simulink model "Nieliniowy"  (R2018a)
settings: Solver=ode45  StartTime=0.0  StopTime=200  RelTol=1e-3  AbsTol=1e-6  EnableMultiTasking=on
values from neighbouring files (symbols this model uses):
  A1 = 3500    [ZbiorniczkiLiniowe.m]
  A2 = 2000    [ZbiorniczkiLiniowe.m]
  Aw1 = 0.1 * A1    (= 350)    [ZbiorniczkiLiniowe.m]
  Aw2 = 0.1 * A2    (= 200)    [ZbiorniczkiLiniowe.m]
  df1 = 200    [ZbiorniczkiLiniowe.m]
  f1 = wektorf1(i)    [ZbiorniczkiLiniowe.m]
  g = 10    [ZbiorniczkiLiniowe.m]
  h1 = (f1/a1)+(f1+df2)/a2    [ZbiorniczkiLiniowe.m]
  h2 = (f1+df2)/a2    [ZbiorniczkiLiniowe.m]
  t1 = 40    [ZbiorniczkiLiniowe.m]
settings Model: Creator=LAB320-1552  LastModifiedBy=johnb
settings SolverCC: AutoScaleAbsTol=off
settings DataIOCC: LimitDataPoints=on  SaveFormat=Array
settings OptimizationCC: LifeSpan=inf
settings DebuggingCC: UnderspecifiedInitializationDetection=Classic  MergeDetectMultiDrivingBlocksExec=none  StateNameClashWarn=warning  StrictBusMsg=ErrorOnBusTreatedAsVector  SFUnexpectedBacktrackingDiag=warning  SFNoUnconditionalDefaultTransitionDiag=warning  SFExecutionAtInitializationDiag=none
settings HardwareCC: ProdBitPerPointer=32  ProdBitPerSizeT=32  ProdBitPerPtrDiffT=32  ProdLargestAtomicFloat=None  ProdIntDivRoundTo=Undefined  ProdEndianess=Unspecified  ProdWordSize=32  ProdHWDeviceType=32-bit Generic
settings ModelReferenceCC: PropagateSignalLabelsOutOfModel=off
settings CodeAppCC: StateflowObjectComments=on
settings GRTTargetCC: TargetLangStandard=C89/C90 (ANSI)  GeneratePreprocessorConditionals=Disable all
settings ConfigComp: CovMetricSettings=dw  CovHtmlReporting=on  CovSaveCumulativeToWorkspaceVar=on  CovSaveSingleToWorkspaceVar=on  CovExternalEMLEnable=off

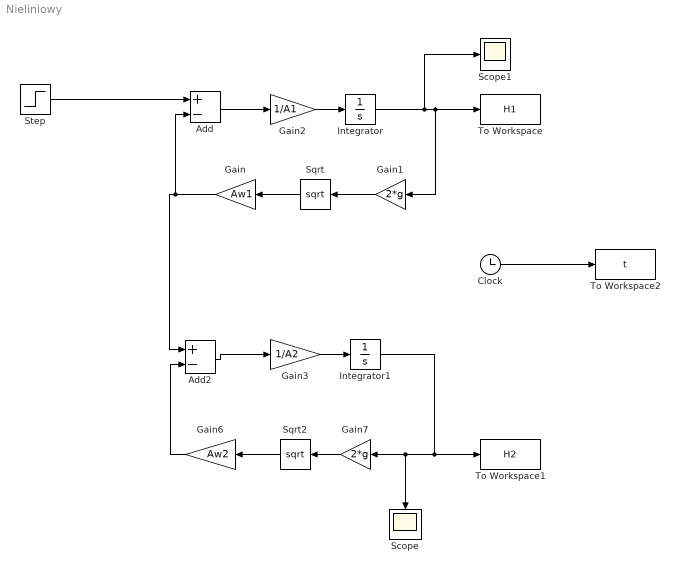
== system Nieliniowy ==
  Add : Sum  Inputs=+-
  Add2 : Sum  Inputs=+-
  Clock : Clock
  Gain : Gain  Gain=Aw1
  Gain1 : Gain  Gain=2*g
  Gain2 : Gain  Gain=1/A1
  Gain3 : Gain  Gain=1/A2
  Gain6 : Gain  Gain=Aw2
  Gain7 : Gain  Gain=2*g
  Integrator : Integrator  InitialCondition=h1
  Integrator1 : Integrator  InitialCondition=h2
  Scope : Scope
  Scope1 : Scope
  Sqrt : Sqrt  SaturateOnIntegerOverflow=on
  Sqrt2 : Sqrt  SaturateOnIntegerOverflow=on
  Step : Step  Time=t1  Before=f1  After=f1+df1  SampleTime=0
  To Workspace : ToWorkspace  VariableName=H1  SampleTime=-1
  To Workspace1 : ToWorkspace  VariableName=H2  SampleTime=-1
  To Workspace2 : ToWorkspace  VariableName=t  SampleTime=-1
  wires:
  Step/1 -> Add/1
  Add/1 -> Gain2/1
  Gain2/1 -> Integrator/1
  Gain1/1 -> Sqrt/1
  Sqrt/1 -> Gain/1
  Gain/1 -> Add/2, Add2/1
  Integrator/1 -> Scope1/1, Gain1/1, To Workspace/1
  Add2/1 -> Gain3/1
  Gain3/1 -> Integrator1/1
  Integrator1/1 -> Scope/1, Gain7/1, To Workspace1/1
  Gain7/1 -> Sqrt2/1
  Sqrt2/1 -> Gain6/1
  Clock/1 -> To Workspace2/1
  Gain6/1 -> Add2/2
